simulink model "Bayoumi_WK10_MDS_legacy"  (R2021a)
settings: Solver=VariableStepAuto  StartTime=0.0  StopTime=50  RelTol=1e-3
values from neighbouring files (symbols this model uses):
  b = 10    [PARA.mat]
  g = 9.8    [PARA.mat]
  k = 10    [PARA.mat]
  m = 10    [PARA.mat]
  SMD_D = 12    [PARA.mat]
  SMD_I = 10    [PARA.mat]
  SMD_P = 11    [PARA.mat]
libraries: fuzblock x1, pid_lib x1
settings Model: OrderedModelArguments=off  Creator=mluser  LastModifiedBy=Ahmed
settings DebuggingCC: UnconnectedInputMsg=none  UnconnectedOutputMsg=none  UnconnectedLineMsg=none
settings ModelReferenceCC: EnableRefExpFcnMdlSchedulingChecks=off
settings RTWCC: Description=Generic Real-Time Target  DLArmComputeVersion=20.02.1

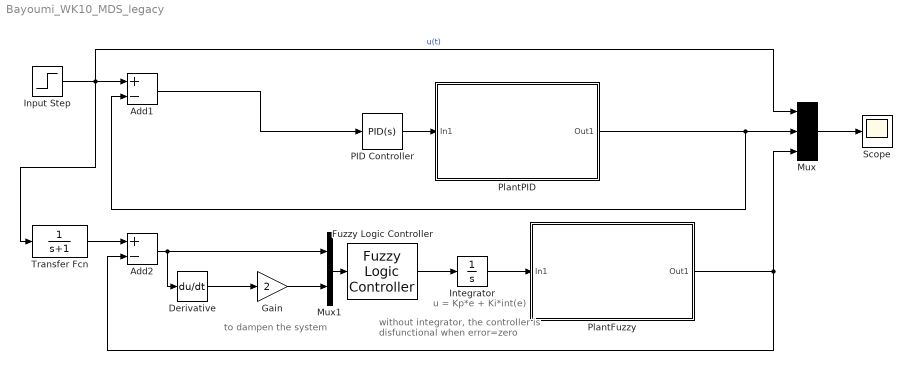
== system Bayoumi_WK10_MDS_legacy ==
  note: to dampen the system
  note: without integrator, the controller is disfunctional when error=zero
  note: u = Kp*e + Ki*int(e)
  Add1 : Sum  Inputs=+-
  Add2 : Sum  Inputs=+-
  Derivative : Derivative
  Fuzzy Logic Controller : fuzblock/Fuzzy Logic  Controller  FIS=fuzzylogic  OutputSampleNumber=101  DataType=double  FuzzifiedInputs=off  RuleFiringStrengths=off  RuleOutputs=off  AggregatedOutputs=off  SimulateUsing=Code generation  OutOfRangeInputValueMessage=warning  NoRuleFiredMessage=warning  EmptyOutputFuzzySetMessage=warning
  Gain : Gain  Gain=2
  Input Step : Step  Time=10  After=5  SampleTime=0
  Integrator : Integrator
  Mux : Mux  Inputs=3
      settings: DisplayOption=signals
  Mux1 : Mux  Inputs=2
  PID Controller : pid_lib/PID Controller  Controller=PID  Form=Parallel  TimeDomain=Continuous-time  UseExternalTs=off  SampleTime=-1  IntegratorMethod=Forward Euler  FilterMethod=Forward Euler  ControllerParametersSource=internal  P=SMD_P  I=SMD_I  D=SMD_D  UseFilter=on  N=100  TunerSelectOption=Frequency Response Based  InitialConditionSource=internal  InitialConditionForIntegrator=0  InitialConditionForFilter=0  DifferentiatorICPrevScaledInput=0  ExternalReset=none  TrackingMode=off  Kt=1  LimitOutput=off  SatLimitsSource=internal  UpperSaturationLimit=inf  LowerSaturationLimit=-inf  LinearizeAsGain=on  AntiWindupMode=none  Kb=1  POutMin=[]  POutMax=[]  IOutMin=[]  IOutMax=[]  DOutMin=[]  DOutMax=[]  NOutMin=[]  NOutMax=[]  SumOutMin=[]  SumOutMax=[]  SaturationOutMin=[]  SaturationOutMax=[]  PParamMin=[]  PParamMax=[]  IParamMin=[]  IParamMax=[]  DParamMin=[]  DParamMax=[]  NParamMin=[]  NParamMax=[]  KbParamMin=[]  KbParamMax=[]  KtParamMin=[]  KtParamMax=[]  KbOutMin=[]  KbOutMax=[]  KtOutMin=[]  KtOutMax=[]  IntegratorOutMin=[]  IntegratorOutMax=[]  FilterOutMin=[]  FilterOutMax=[]  SumI1OutMin=[]  SumI1OutMax=[]  SumI2OutMin=[]  SumI2OutMax=[]  SumI3OutMin=[]  SumI3OutMax=[]  SumI4OutMin=[]  SumI4OutMax=[]  SumDOutMin=[]  SumDOutMax=[]  DifferentiatorOutMin=[]  DifferentiatorOutMax=[]  FilterDiffOutCoefMin=[]  FilterDiffOutCoefMax=[]  ReciprocalOutMin=[]  ReciprocalOutMax=[]  SumDenOutMin=[]  SumDenOutMax=[]  SumNumOutMin=[]  SumNumOutMax=[]  DivideOutMin=[]  DivideOutMax=[]  UdiffTsProdOutMin=[]  UdiffTsProdOutMax=[]  NTsProdOutMin=[]  NTsProdOutMax=[]  UintegralTsProdOutMin=[]  UintegralTsProdOutMax=[]  UngainTsProdOutMin=[]  UngainTsProdOutMax=[]  IntegratorContinuousStateAttributes=''  IntegratorStateMustResolveToSignalObject=off  IntegratorRTWStateStorageClass=Auto  FilterContinuousStateAttributes=''  FilterStateMustResolveToSignalObject=off  FilterRTWStateStorageClass=Auto  ParallelPVariant=InternalParameters  IdealPVariant=Disabled  IVariant=InternalParameters  DVariant=InternalParameters  IntegratorVariant=Continuous  SatVariant=Disabled  AWVariant=Passthrough  PCopyVariant=Disabled  TRVariant=Disabled  FdbkBlocksVariant=Forward  IdealPFdbkVariant=Disabled  SatFdbkVariant=Disabled  DerivativeFilterVariant=ContFilter  NVariant=InternalParameters  NCopyVariant=Disabled  FilterICVariant=InternalICsFilter  IntegratorICVariant=InternalICs  ExternalResetVariant=Disabled  TRSumVariant=Passthrough  SumFdbkVariant=Disabled  SumVariant=Sum_PID  TsampFilterVariant=InternalTs  TsampNgainVariant=Passthrough  TsampIntegralVariant=Passthrough  ExternalSaturationOutDataTypeStr=Inherit: Same as second input
  PlantFuzzy : Subsystem
  PlantPID : Subsystem
  Scope : Scope
  Transfer Fcn : TransferFcn  Denominator=[1 1]
  wires:
  Input Step/1 -> Transfer Fcn/1, Add1/1, Mux/1  "u(t)"
  Mux/1 -> Scope/1
  Add1/1 -> PID Controller/1
  PID Controller/1 -> PlantPID/1(In1)
  PlantPID/1(Out1) -> Add1/2, Mux/2
  PlantFuzzy/1(Out1) -> Mux/3, Add2/2
  Mux1/1 -> Fuzzy Logic Controller/1
  Add2/1 -> Derivative/1, Mux1/1
  Derivative/1 -> Gain/1
  Fuzzy Logic Controller/1 -> Integrator/1
  Transfer Fcn/1 -> Add2/1
  Integrator/1 -> PlantFuzzy/1(In1)
  Gain/1 -> Mux1/2

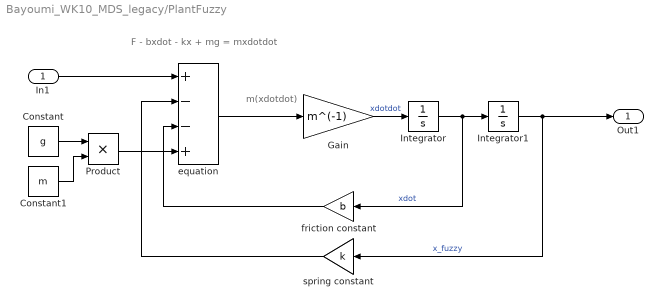
== system Bayoumi_WK10_MDS_legacy/PlantFuzzy ==
  note: m(xdotdot)
  note: F - bxdot - kx + mg = mxdotdot
  In1 : Inport
  Constant : Constant  Value=g
  Constant1 : Constant  Value=m
  Gain : Gain  Gain=m^(-1)
  Integrator : Integrator
  Integrator1 : Integrator
  Product : Product
  equation : Sum  Inputs=+--+
  friction constant : Gain  Gain=b
  spring constant : Gain  Gain=k
  Out1 : Outport
  wires:
  equation/1 -> Gain/1
  Constant/1 -> Product/1
  Integrator1/1 -> Out1/1, spring constant/1  "x_fuzzy"
  friction constant/1 -> equation/3
  spring constant/1 -> equation/2
  Product/1 -> equation/4
  Constant1/1 -> Product/2
  Integrator/1 -> friction constant/1, Integrator1/1  "xdot"
  Gain/1 -> Integrator/1  "xdotdot"
  In1/1 -> equation/1

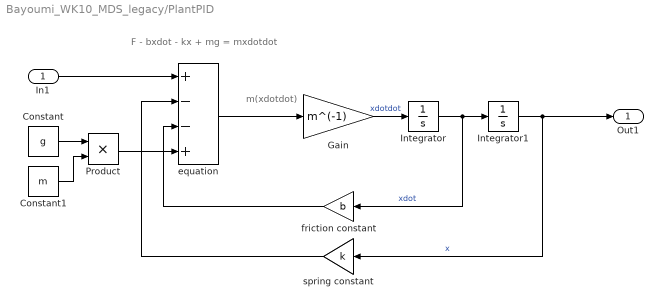
== system Bayoumi_WK10_MDS_legacy/PlantPID ==
  note: m(xdotdot)
  note: F - bxdot - kx + mg = mxdotdot
  In1 : Inport
  Constant : Constant  Value=g
  Constant1 : Constant  Value=m
  Gain : Gain  Gain=m^(-1)
  Integrator : Integrator
  Integrator1 : Integrator
  Product : Product
  equation : Sum  Inputs=+--+
  friction constant : Gain  Gain=b
  spring constant : Gain  Gain=k
  Out1 : Outport
  wires:
  equation/1 -> Gain/1
  Constant/1 -> Product/1
  Integrator1/1 -> Out1/1, spring constant/1  "x"
  friction constant/1 -> equation/3
  spring constant/1 -> equation/2
  Product/1 -> equation/4
  Constant1/1 -> Product/2
  Integrator/1 -> friction constant/1, Integrator1/1  "xdot"
  Gain/1 -> Integrator/1  "xdotdot"
  In1/1 -> equation/1
